simulink model "model2"  (R2012b)
settings: Solver=ode3  StartTime=0.0  StopTime=inf  FixedStep=0.001  RelTol=1e-3
undefined symbols (not defined in the file): HIL
libraries: quarc_library x5
settings Model: SimulationMode=external  ExtModeTrigDuration=50000  Creator=ray.xu  LastModifiedBy=paichihyun
settings SolverCC: PositivePriorityOrder=on
settings DataIOCC: LimitDataPoints=off
settings RTWCC: SystemTargetFile=quarc_win64.tlc  TemplateMakefile=quarc_default_tmf  Description=QUARC Win64 Target  ProcessScript=quarc_win64_make_rtw_hook
settings STFCustomTargetCC: TargetPreCompLibLocation=C:\PROGRA~3\QUARC\lib\2012b\win64\release  CodeReplacementLibrary=ANSI_C  GeneratePreprocessorConditionals=Disable all  CombineOutputUpdateFcns=on  GRTInterface=off  SystemTargetFile=quarc_win64.tlc
settings GRTTargetCC: TargetPreCompLibLocation=C:\PROGRA~3\QUARC\lib\2012b\win64\release  ParMdlRefBuildCompliant=off  CompOptLevelCompliant=off  ConcurrentExecutionCompliant=off  MatFileLogging=off  ExtMode=on  ExtModeMexFile=quarc_comm
settings ConfigurationSet: Description=SimMechanics 2G

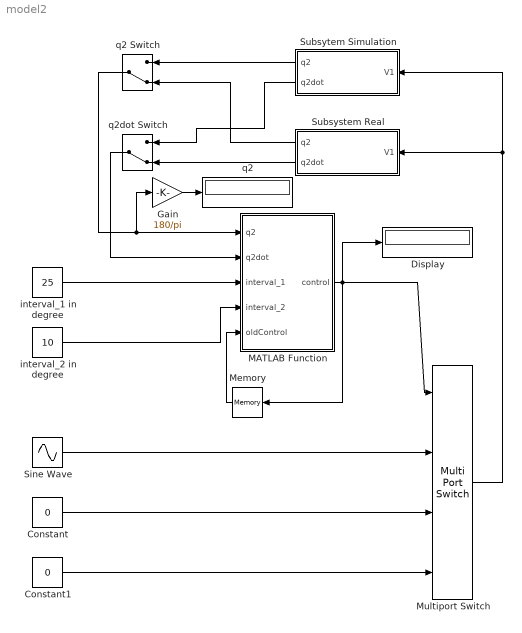
== system model2 ==
  Constant : Constant  Value=0
  Constant1 : Constant  Value=0
  Display : Display
  Gain : Gain  Gain=180/pi
  MATLAB Function : MATLAB Function  TreatAsAtomicUnit=on
  Memory : Memory  X0=1
  Multiport Switch : MultiPortSwitch
  Sine Wave : Sin  Amplitude=0  Frequency=0  SampleTime=0
  Subsystem Real : Subsystem
  Subsytem Simulation : Subsystem
  interval_1 in degree : Constant  Value=25
  interval_2 in degree : Constant  Value=10
  q2 : Display
  q2 Switch : ManualSwitch  CurrentSetting=0
  q2dot Switch : ManualSwitch  CurrentSetting=0
  wires:
  Constant/1 -> Multiport Switch/3
  Constant1/1 -> Multiport Switch/4
  Multiport Switch/1 -> Subsystem Real/1(V1), Subsytem Simulation/1(V1)
  Subsytem Simulation/2(q2dot) -> q2dot Switch/1
  Subsystem Real/1(q2) -> q2 Switch/2
  Subsystem Real/2(q2dot) -> q2dot Switch/2
  Subsytem Simulation/1(q2) -> q2 Switch/1
  q2 Switch/1 -> Gain/1, MATLAB Function/1(q2)
  q2dot Switch/1 -> MATLAB Function/2(q2dot)
  Sine Wave/1 -> Multiport Switch/2
  interval_1 in degree/1 -> MATLAB Function/3(interval_1)
  interval_2 in degree/1 -> MATLAB Function/4(interval_2)
  MATLAB Function/1(control) -> Display/1, Multiport Switch/1, Memory/1
  Memory/1 -> MATLAB Function/5(oldControl)
  Gain/1 -> q2/1

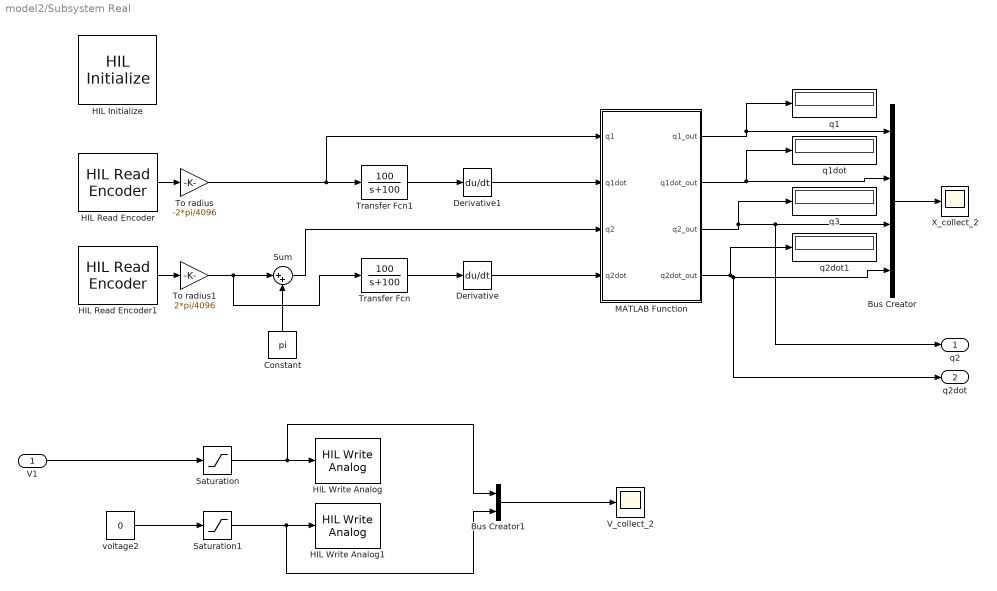
== system model2/Subsystem Real ==
  V1 : Inport
  Bus Creator : BusCreator
  Bus Creator1 : BusCreator  Inputs=2
  Constant : Constant  Value=pi
  Derivative : Derivative
  Derivative1 : Derivative
  HIL Initialize : quarc_library/Data Acquisition/Generic/Configuration/HIL Initialize  Priority=-99  object_name=HIL-1  board_type=q2_usb  board_number=0  board_options=d0=digital;d1=digital;led=auto;update_rate=normal;decimation=1  exclusive=off  active=off  hardware_clocks=[0]  clock_modes=[]  initial_clock_frequencies=[]  set_clock_params_at_start=off  set_clock_params_at_switch_in=off  set_clock_frequencies_at_start=off  set_clock_frequencies_at_switch_in=off  analog_input_channels=[0:1]  analog_input_maximums=10  analog_input_minimums=-10  set_analog_input_params_at_start=on  set_analog_input_params_at_switch_in=off  analog_output_channels=[0:1]  analog_output_maximums=10  analog_output_minimums=-10  initial_analog_outputs=[0]  final_analog_outputs=[0]  watchdog_analog_outputs=0  set_analog_output_params_at_start=on  set_analog_output_params_at_switch_in=off  set_analog_outputs_at_start=on  set_analog_outputs_at_switch_in=off  set_analog_outputs_at_terminate=on  set_analog_outputs_at_switch_out=off  set_analog_outputs_on_watchdog=off  digital_input_channels=[]  digital_output_channels=[]  digital_output_configuration=[]  initial_digital_outputs=[1]  final_digital_outputs=[1]  watchdog_digital_outputs=[1]  set_digital_output_params_at_start=off  set_digital_output_params_at_switch_in=off  set_digital_outputs_at_start=on  set_digital_outputs_at_switch_in=off  set_digital_outputs_at_terminate=on  set_digital_outputs_at_switch_out=off  set_digital_outputs_on_watchdog=off  encoder_channels=[0:1]  quadrature=[4]  encoder_filter_frequency=[]  initial_encoder_counts=[0]  set_encoder_params_at_start=on  set_encoder_params_at_switch_in=off  set_encoder_counts_at_start=on  set_encoder_counts_at_switch_in=off  pwm_channels=[]  pwm_modes=[0]  pwm_frequency=1/0.020  pwm_configuration=[]  pwm_alignment=[]  pwm_polarity=[]  pwm_leading_deadband=[]  pwm_trailing_deadband=[]  initial_pwm_outputs=[0]  final_pwm_outputs=[0]  watchdog_pwm_outputs=[0]  set_pwm_params_at_start=on  set_pwm_params_at_switch_in=off  set_pwm_outputs_at_start=on  set_pwm_outputs_at_switch_in=off  set_pwm_outputs_at_terminate=on  set_pwm_outputs_at_switch_out=off  set_pwm_outputs_on_watchdog=off  other_output_channels=[]  initial_other_outputs=[]  final_other_outputs=[]  watchdog_other_outputs=[]  set_other_outputs_at_start=off  set_other_outputs_at_switch_in=off  set_other_outputs_at_terminate=off  set_other_outputs_at_switch_out=off  set_other_outputs_on_watchdog=off
  HIL Read Encoder : quarc_library/Data Acquisition/Generic/Immediate I//O/HIL Read Encoder  object_name=HIL-1  channels=0  sample_time=qc_get_step_size  active=on  vector_output=off  data_type_mode=Inherit via back propagation  data_type=double
  HIL Read Encoder1 : quarc_library/Data Acquisition/Generic/Immediate I//O/HIL Read Encoder  object_name=HIL-1  channels=1  sample_time=qc_get_step_size  active=on  vector_output=off  data_type_mode=Inherit via back propagation  data_type=double
  HIL Write Analog : quarc_library/Data Acquisition/Generic/Immediate I//O/HIL Write Analog  object_name=HIL-1  channels=0  sample_time=-1  active=off  vector_input=off
  HIL Write Analog1 : quarc_library/Data Acquisition/Generic/Immediate I//O/HIL Write Analog  object_name=HIL-1  channels=1  sample_time=-1  active=off  vector_input=off
  MATLAB Function : MATLAB Function  TreatAsAtomicUnit=on
  Saturation : Saturate  UpperLimit=10  LowerLimit=-10
  Saturation1 : Saturate  UpperLimit=10  LowerLimit=-10
  Sum : Sum  Inputs=|++
  To radius : Gain  Gain=-2*pi/4096
  To radius1 : Gain  Gain=2*pi/4096
  Transfer Fcn : TransferFcn  Numerator=[100]  Denominator=[1 100]
  Transfer Fcn1 : TransferFcn  Numerator=[100]  Denominator=[1 100]
  V_collect_2 : Scope
      settings: SaveName=V_collect_  SampleInput=on  SampleTime=0.001
  "X_collect_2 " : Scope
      settings: SaveName=X_collect_  SampleInput=on  SampleTime=0.001
  q1 : Display
  q1dot : Display
  q2dot1 : Display
  q3 : Display
  voltage2 : Constant  Value=0
  q2 : Outport
  q2dot : Outport  Port=2
  wires:
  Transfer Fcn/1 -> Derivative/1
  HIL Read Encoder/1 -> To radius/1
  HIL Read Encoder1/1 -> To radius1/1
  Constant/1 -> Sum/2
  To radius1/1 -> Transfer Fcn/1, Sum/1
  Transfer Fcn1/1 -> Derivative1/1
  To radius/1 -> MATLAB Function/1(q1), Transfer Fcn1/1
  Sum/1 -> MATLAB Function/3(q2)
  Derivative/1 -> MATLAB Function/4(q2dot)
  Derivative1/1 -> MATLAB Function/2(q1dot)
  Saturation/1 -> Bus Creator1/1, HIL Write Analog/1
  Saturation1/1 -> Bus Creator1/2, HIL Write Analog1/1
  voltage2/1 -> Saturation1/1
  Bus Creator1/1 -> V_collect_2/1
  V1/1 -> Saturation/1
  MATLAB Function/1(q1_out) -> Bus Creator/1, q1/1
  MATLAB Function/3(q2_out) -> q2/1, Bus Creator/3, q3/1
  MATLAB Function/4(q2dot_out) -> q2dot1/1, Bus Creator/4, q2dot/1
  MATLAB Function/2(q1dot_out) -> q1dot/1, Bus Creator/2
  Bus Creator/1 -> "X_collect_2 "/1

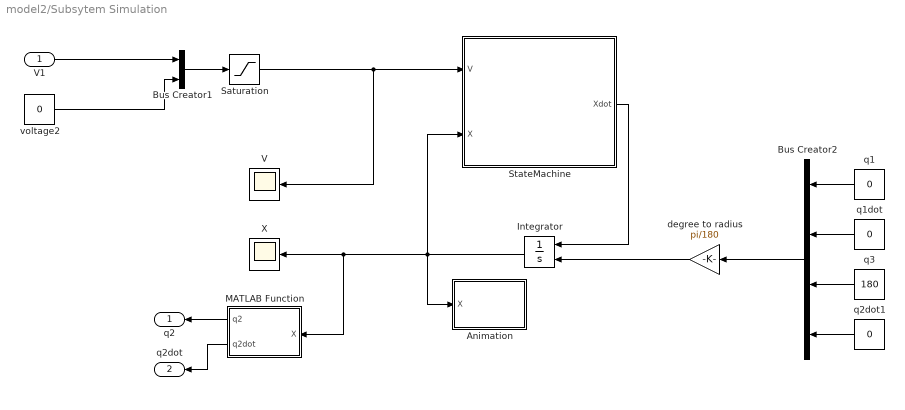
== system model2/Subsytem Simulation ==
  V1 : Inport
  Animation : MATLAB Function  TreatAsAtomicUnit=on
  Bus Creator1 : BusCreator  Inputs=2
  Bus Creator2 : BusCreator
  Integrator : Integrator  InitialConditionSource=external
  MATLAB Function : MATLAB Function  TreatAsAtomicUnit=on
  Saturation : Saturate  UpperLimit=10  LowerLimit=-10
  StateMachine : MATLAB Function  TreatAsAtomicUnit=on
  V : Scope
      settings: SaveName=V_collect  MaxDataPoints=10800
  X : Scope
      settings: SaveName=X_collect  MaxDataPoints=10800
  degree to radius : Gain  Gain=pi/180
  q1 : Constant  Value=0
  q1dot : Constant  Value=0
  q2dot1 : Constant  Value=0
  q3 : Constant  Value=180
  voltage2 : Constant  Value=0
  q2 : Outport
  q2dot : Outport  Port=2
  wires:
  voltage2/1 -> Bus Creator1/2
  Bus Creator1/1 -> Saturation/1
  StateMachine/1(Xdot) -> Integrator/1
  Integrator/1 -> Animation/1(X), MATLAB Function/1(X), X/1, StateMachine/2(X)
  q1/1 -> Bus Creator2/1
  q1dot/1 -> Bus Creator2/2
  q3/1 -> Bus Creator2/3
  q2dot1/1 -> Bus Creator2/4
  Bus Creator2/1 -> degree to radius/1
  degree to radius/1 -> Integrator/2
  MATLAB Function/1(q2) -> q2/1
  MATLAB Function/2(q2dot) -> q2dot/1
  Saturation/1 -> V/1, StateMachine/1(V)
  V1/1 -> Bus Creator1/1

== matlab function model2/Subsytem Simulation/Animation ==
  data: X input
function Animation(X)

theta1 = X(1);
theta2 = X(3);
% Sphere();
L1 = 6;
L2 = 2;
P0_Org=[0;0;0;1];
P1_Org=[0;0;-1;1];
P2_Org=[0;6;-1;1];
P3_Org=[0;6;0;1];
P4_Org=[0;8;0;1];
P5_Org=[0;12;0;1];

% theta1 = theta1 * pi / 180;
% theta2 = theta2 * pi / 180;

T01 = [cos(theta1),-sin(theta1),0,0;sin(theta1),cos(theta1),0,0;0,0,1,0;0,0,0,1];
P1 = T01 * P1_Org;
P2 = T01 * P2_Org;
P3 = T01 * P3_Org;
P4 = T01 * P4_Org;
T12 = [cos(theta2),-sin(theta2),0,0;0,0,-1,(L1+L2);sin(theta2),cos(theta2),0,0;0,0,0,1];
P5 = T01 * T12 * P5_Org;

plot3([P0_Org(1),P1(1),P2(1),P3(1),P4(1),P5(1)], [P0_Org(2),P1(2),P2(2),P3(2),P4(2),P5(2)], [P0_Org(3),P1(3),P2(3),P3(3),P4(3),P5(3)],'-o');
title('Robot Representation'); grid on;xlim([-10 10]);ylim([-10 10]);zlim([-10 10]);xlabel('x');ylabel('y');zlabel('z');
% drawnow
end

== matlab function model2/MATLAB Function ==
  data: q2 input; control output; q2dot input; interval_1 input; interval_2 input; oldControl input
function control  = control_func(q2, q2dot, interval_1, interval_2, oldControl)
% interval_1 = 25;
% interval_2 = 10;
point_a = (interval_1)*pi/180;
point_b = (360-interval_1)*pi/180;
point_c = (180-interval_2)*pi/180;
point_d = (180+interval_2)*pi/180;


if(q2 < point_a || q2 > point_b)
    currentState = 3;
elseif(q2 > point_c && q2 < point_d)
    currentState = 1;
else
    currentState = 2;
end

if(oldControl == 1 && currentState == 3 )
    control = 3;
elseif oldControl == 2 && currentState == 1
    control = 1;
elseif oldControl == 3 && currentState == 2
    control = 2;
else
    control = oldControl;
end
end

== matlab function model2/Subsytem Simulation/StateMachine ==
  data: V input; Xdot output; X input
function Xdot  =StateMachine(V, X)

% J1=0.0012;
% m2=0.127;
% l1_l2=0.2;
% l2=0.3;
% lc2=0.15;
% beta1=0.015;
% beta2=0.002;
% Ra=2.6;
% kt=0.00768;
% kv=0.00768;
% kr=70;
% 
% theta1=(J1+m2*l1_l2^2)*Ra/(kr*kt);
% theta2=(m2*l2^2/3)*Ra/(kr*kt);
% theta3=(m2*l1_l2*l2/2)*Ra/(kr*kt);

% theta4=(m2*lc2)*Ra/(kr*kt);
% theta5=beta1*Ra/(kr*kt) + kr*kv;
% theta6=beta2*Ra/(kr*kt);

q1=X(1);
q1dot=X(2);
q2=X(3);
q2dot=X(4);

theta1=0.030372023809524;
theta2=0.018426339285714;
theta3=0.018426339285714;
theta4=0.092131696428571;
theta5=0.610144642857143;
theta6=0.009672619047619;

m11=theta1+theta2*sin(q2)^2;
m12=theta3*cos(q2);
m21=theta3*cos(q2);
m22=theta2;
c11=2*theta2*sin(q2)*cos(q2)*q2dot;
c12=-theta3*sin(q2)*q2dot;
c21=-theta2*sin(q2)*cos(q2)*q1dot;
c22=0;
f1=theta5*q1dot;
f2=theta6*q2dot;                           
g=9.8;
g1=0;
g2=-theta4*g*sin(q2);

M=[m11,m12;m21,m22];
C=[c11,c12;c21,c22];
F=[f1;f2];
G=[g1;g2];
qdot=[q1dot;q2dot];

qdotdot=M\(V-C*qdot-F-G); 
Xdot=[q1dot,qdotdot(1),q2dot,qdotdot(2)];
Q=[q1;q2];
end

== matlab function model2/Subsytem Simulation/MATLAB Function ==
  data: X input; q2 output; q2dot output
function [q2, q2dot] = extract(X)
%#codegen
q2 = X(3);
q2dot = X(4);
end

== matlab function model2/Subsystem Real/MATLAB Function ==
  data: q1 input; q1_out output; q1dot input; q2 input; q2dot input; q1dot_out output; q2_out output; q2dot_out output
function [q1_out, q1dot_out, q2_out, q2dot_out] = mod_2pi(q1, q1dot, q2, q2dot)
q1_out = mod(q1, 2*pi);
q1dot_out = q1dot;
q2_out = mod(q2, 2*pi);
q2dot_out = q2dot;
end
